simulink model "model_cnn"  (R2020a)
settings: Solver=VariableStepAuto  StartTime=0.0  StopTime=1e6/fs  RelTol=1e-3
PreLoadFcn:
  | setup_imports;
  | %dense2_numerictype = fixdt(1,18,10);
  | %conv1_numerictype = fixdt(1,18,21);
InitFcn:
  | % Intermediate signal dimensions
  | input_dim = [1, 2, 128];
  | layer1_dim = hInterConvLayerDims([1,3,1,64],input_dim,1); % dims : [C,H,W]
  | layer2_dim = hInterConvLayerDims([2,3,64,16],layer1_dim,1);% dims : [C,H,W]
  | layer3_dim = [1,128];
  | 
  | % Conv Layer 1 dimensions
  | conv1_dims = struct(...
  |     'input_dim',    input_dim,...       input_dim = C,H,W
  |     'filter_dim',   [1, 3, 1, 64],...  filter_dim = K,J,C,N
  |     'stride',       1,...
  |     'row_output',   3,...
  |     'output_dim',   layer1_dim);
  | 
  | % Conv Layer 2 dimensions
  | conv2_dims = struct(...
  |     'input_dim',    layer1_dim,...      input = C,H.W
  |     'filter_dim',   [2, 3, 64, 16],...  filter_dim = K,J,C,N
  |     'stride',       1,...
  |     'row_output',   2*3*64,...
  |     'output_dim',   layer2_dim);
  | 
  | % Dense Layer 1 dimensions
  | dense1_dims = struct(...
  |     'input_dim',    layer2_dim,...      input = C,H,W
  |     'weight_dim',   [1984, 128],...     weight_dim = H,W
  |     'output_dim',   layer3_dim);
  | 
  | % Load saved weights and input
  | setup_imports;
  | 
  | fs = 128e6;
  | fs_axi = 100e6;
  | R = 32;
values from neighbouring files (symbols this model uses):
  datatypeInput = X_test.numerictype    [setup_imports.m]
  gemm_wconv1 = fi(hInterleaveFilters(Wconv1),1,16)    [setup_imports.m]
  gemm_wconv2 = fi(hInterleaveFilters(Wconv2),1,16)    [setup_imports.m]
  wdense1 = fi(Wdense1,1,16)    [setup_imports.m]
  wdense2 = fi(Wdense2,1,16)    [setup_imports.m]
undefined symbols (not defined in the file or in its folder): ltehdlRAMinitPO2
libraries: hdlsllib x1022, dspsigops x3, dspsrcs4 x2
(part 3 of 23)

== system model_cnn/HDL CNN Model/Conv Layer 1/Layer 1 Mat-Vec Multiplier/Weight Storage13 ==
  count_Weights : Inport
  Constant : Constant  Value=0  OutDataTypeStr=gemm_wconv1.numerictype  SampleTime=-1
  Constant1 : Constant  Value=false  SampleTime=-1
  Single Port RAM System : hdlsllib/HDL RAMs/Single Port RAM System  RAMType=Single port  WriteOutputValue=New data  RAMInitialValue=[gemm_wconv1(dim,:),zeros(1,4-3)]  SimulateUsing=Code generation
      settings: SourceProductBaseCode=SL
  Out1 : Outport
  wires:
  Single Port RAM System/1 -> Out1/1
  Constant/1 -> Single Port RAM System/1
  Constant1/1 -> Single Port RAM System/3
  count_Weights/1 -> Single Port RAM System/2

== system model_cnn/HDL CNN Model/Conv Layer 1/Layer 1 Mat-Vec Multiplier/Weight Storage14 ==
  count_Weights : Inport
  Constant : Constant  Value=0  OutDataTypeStr=gemm_wconv1.numerictype  SampleTime=-1
  Constant1 : Constant  Value=false  SampleTime=-1
  Single Port RAM System : hdlsllib/HDL RAMs/Single Port RAM System  RAMType=Single port  WriteOutputValue=New data  RAMInitialValue=[gemm_wconv1(dim,:),zeros(1,4-3)]  SimulateUsing=Code generation
      settings: SourceProductBaseCode=SL
  Out1 : Outport
  wires:
  Single Port RAM System/1 -> Out1/1
  Constant/1 -> Single Port RAM System/1
  Constant1/1 -> Single Port RAM System/3
  count_Weights/1 -> Single Port RAM System/2

== system model_cnn/HDL CNN Model/Conv Layer 1/Layer 1 Mat-Vec Multiplier/Weight Storage15 ==
  count_Weights : Inport
  Constant : Constant  Value=0  OutDataTypeStr=gemm_wconv1.numerictype  SampleTime=-1
  Constant1 : Constant  Value=false  SampleTime=-1
  Single Port RAM System : hdlsllib/HDL RAMs/Single Port RAM System  RAMType=Single port  WriteOutputValue=New data  RAMInitialValue=[gemm_wconv1(dim,:),zeros(1,4-3)]  SimulateUsing=Code generation
      settings: SourceProductBaseCode=SL
  Out1 : Outport
  wires:
  Single Port RAM System/1 -> Out1/1
  Constant/1 -> Single Port RAM System/1
  Constant1/1 -> Single Port RAM System/3
  count_Weights/1 -> Single Port RAM System/2

== system model_cnn/HDL CNN Model/Conv Layer 1/Layer 1 Mat-Vec Multiplier/Weight Storage16 ==
  count_Weights : Inport
  Constant : Constant  Value=0  OutDataTypeStr=gemm_wconv1.numerictype  SampleTime=-1
  Constant1 : Constant  Value=false  SampleTime=-1
  Single Port RAM System : hdlsllib/HDL RAMs/Single Port RAM System  RAMType=Single port  WriteOutputValue=New data  RAMInitialValue=[gemm_wconv1(dim,:),zeros(1,4-3)]  SimulateUsing=Code generation
      settings: SourceProductBaseCode=SL
  Out1 : Outport
  wires:
  Single Port RAM System/1 -> Out1/1
  Constant/1 -> Single Port RAM System/1
  Constant1/1 -> Single Port RAM System/3
  count_Weights/1 -> Single Port RAM System/2

== system model_cnn/HDL CNN Model/Conv Layer 1/Layer 1 Mat-Vec Multiplier/Weight Storage17 ==
  count_Weights : Inport
  Constant : Constant  Value=0  OutDataTypeStr=gemm_wconv1.numerictype  SampleTime=-1
  Constant1 : Constant  Value=false  SampleTime=-1
  Single Port RAM System : hdlsllib/HDL RAMs/Single Port RAM System  RAMType=Single port  WriteOutputValue=New data  RAMInitialValue=[gemm_wconv1(dim,:),zeros(1,4-3)]  SimulateUsing=Code generation
      settings: SourceProductBaseCode=SL
  Out1 : Outport
  wires:
  Single Port RAM System/1 -> Out1/1
  Constant/1 -> Single Port RAM System/1
  Constant1/1 -> Single Port RAM System/3
  count_Weights/1 -> Single Port RAM System/2

== system model_cnn/HDL CNN Model/Conv Layer 1/Layer 1 Mat-Vec Multiplier/Weight Storage18 ==
  count_Weights : Inport
  Constant : Constant  Value=0  OutDataTypeStr=gemm_wconv1.numerictype  SampleTime=-1
  Constant1 : Constant  Value=false  SampleTime=-1
  Single Port RAM System : hdlsllib/HDL RAMs/Single Port RAM System  RAMType=Single port  WriteOutputValue=New data  RAMInitialValue=[gemm_wconv1(dim,:),zeros(1,4-3)]  SimulateUsing=Code generation
      settings: SourceProductBaseCode=SL
  Out1 : Outport
  wires:
  Single Port RAM System/1 -> Out1/1
  Constant/1 -> Single Port RAM System/1
  Constant1/1 -> Single Port RAM System/3
  count_Weights/1 -> Single Port RAM System/2

== system model_cnn/HDL CNN Model/Conv Layer 1/Layer 1 Mat-Vec Multiplier/Weight Storage19 ==
  count_Weights : Inport
  Constant : Constant  Value=0  OutDataTypeStr=gemm_wconv1.numerictype  SampleTime=-1
  Constant1 : Constant  Value=false  SampleTime=-1
  Single Port RAM System : hdlsllib/HDL RAMs/Single Port RAM System  RAMType=Single port  WriteOutputValue=New data  RAMInitialValue=[gemm_wconv1(dim,:),zeros(1,4-3)]  SimulateUsing=Code generation
      settings: SourceProductBaseCode=SL
  Out1 : Outport
  wires:
  Single Port RAM System/1 -> Out1/1
  Constant/1 -> Single Port RAM System/1
  Constant1/1 -> Single Port RAM System/3
  count_Weights/1 -> Single Port RAM System/2

== system model_cnn/HDL CNN Model/Conv Layer 1/Layer 1 Mat-Vec Multiplier/Weight Storage2 ==
  count_Weights : Inport
  Constant : Constant  Value=0  OutDataTypeStr=gemm_wconv1.numerictype  SampleTime=-1
  Constant1 : Constant  Value=false  SampleTime=-1
  Single Port RAM System : hdlsllib/HDL RAMs/Single Port RAM System  RAMType=Single port  WriteOutputValue=New data  RAMInitialValue=[gemm_wconv1(dim,:),zeros(1,4-3)]  SimulateUsing=Code generation
      settings: SourceProductBaseCode=SL
  Out1 : Outport
  wires:
  Single Port RAM System/1 -> Out1/1
  Constant/1 -> Single Port RAM System/1
  Constant1/1 -> Single Port RAM System/3
  count_Weights/1 -> Single Port RAM System/2

== system model_cnn/HDL CNN Model/Conv Layer 1/Layer 1 Mat-Vec Multiplier/Weight Storage20 ==
  count_Weights : Inport
  Constant : Constant  Value=0  OutDataTypeStr=gemm_wconv1.numerictype  SampleTime=-1
  Constant1 : Constant  Value=false  SampleTime=-1
  Single Port RAM System : hdlsllib/HDL RAMs/Single Port RAM System  RAMType=Single port  WriteOutputValue=New data  RAMInitialValue=[gemm_wconv1(dim,:),zeros(1,4-3)]  SimulateUsing=Code generation
      settings: SourceProductBaseCode=SL
  Out1 : Outport
  wires:
  Single Port RAM System/1 -> Out1/1
  Constant/1 -> Single Port RAM System/1
  Constant1/1 -> Single Port RAM System/3
  count_Weights/1 -> Single Port RAM System/2

== system model_cnn/HDL CNN Model/Conv Layer 1/Layer 1 Mat-Vec Multiplier/Weight Storage21 ==
  count_Weights : Inport
  Constant : Constant  Value=0  OutDataTypeStr=gemm_wconv1.numerictype  SampleTime=-1
  Constant1 : Constant  Value=false  SampleTime=-1
  Single Port RAM System : hdlsllib/HDL RAMs/Single Port RAM System  RAMType=Single port  WriteOutputValue=New data  RAMInitialValue=[gemm_wconv1(dim,:),zeros(1,4-3)]  SimulateUsing=Code generation
      settings: SourceProductBaseCode=SL
  Out1 : Outport
  wires:
  Single Port RAM System/1 -> Out1/1
  Constant/1 -> Single Port RAM System/1
  Constant1/1 -> Single Port RAM System/3
  count_Weights/1 -> Single Port RAM System/2

== system model_cnn/HDL CNN Model/Conv Layer 1/Layer 1 Mat-Vec Multiplier/Weight Storage22 ==
  count_Weights : Inport
  Constant : Constant  Value=0  OutDataTypeStr=gemm_wconv1.numerictype  SampleTime=-1
  Constant1 : Constant  Value=false  SampleTime=-1
  Single Port RAM System : hdlsllib/HDL RAMs/Single Port RAM System  RAMType=Single port  WriteOutputValue=New data  RAMInitialValue=[gemm_wconv1(dim,:),zeros(1,4-3)]  SimulateUsing=Code generation
      settings: SourceProductBaseCode=SL
  Out1 : Outport
  wires:
  Single Port RAM System/1 -> Out1/1
  Constant/1 -> Single Port RAM System/1
  Constant1/1 -> Single Port RAM System/3
  count_Weights/1 -> Single Port RAM System/2

== system model_cnn/HDL CNN Model/Conv Layer 1/Layer 1 Mat-Vec Multiplier/Weight Storage23 ==
  count_Weights : Inport
  Constant : Constant  Value=0  OutDataTypeStr=gemm_wconv1.numerictype  SampleTime=-1
  Constant1 : Constant  Value=false  SampleTime=-1
  Single Port RAM System : hdlsllib/HDL RAMs/Single Port RAM System  RAMType=Single port  WriteOutputValue=New data  RAMInitialValue=[gemm_wconv1(dim,:),zeros(1,4-3)]  SimulateUsing=Code generation
      settings: SourceProductBaseCode=SL
  Out1 : Outport
  wires:
  Single Port RAM System/1 -> Out1/1
  Constant/1 -> Single Port RAM System/1
  Constant1/1 -> Single Port RAM System/3
  count_Weights/1 -> Single Port RAM System/2

== system model_cnn/HDL CNN Model/Conv Layer 1/Layer 1 Mat-Vec Multiplier/Weight Storage24 ==
  count_Weights : Inport
  Constant : Constant  Value=0  OutDataTypeStr=gemm_wconv1.numerictype  SampleTime=-1
  Constant1 : Constant  Value=false  SampleTime=-1
  Single Port RAM System : hdlsllib/HDL RAMs/Single Port RAM System  RAMType=Single port  WriteOutputValue=New data  RAMInitialValue=[gemm_wconv1(dim,:),zeros(1,4-3)]  SimulateUsing=Code generation
      settings: SourceProductBaseCode=SL
  Out1 : Outport
  wires:
  Single Port RAM System/1 -> Out1/1
  Constant/1 -> Single Port RAM System/1
  Constant1/1 -> Single Port RAM System/3
  count_Weights/1 -> Single Port RAM System/2

== system model_cnn/HDL CNN Model/Conv Layer 1/Layer 1 Mat-Vec Multiplier/Weight Storage25 ==
  count_Weights : Inport
  Constant : Constant  Value=0  OutDataTypeStr=gemm_wconv1.numerictype  SampleTime=-1
  Constant1 : Constant  Value=false  SampleTime=-1
  Single Port RAM System : hdlsllib/HDL RAMs/Single Port RAM System  RAMType=Single port  WriteOutputValue=New data  RAMInitialValue=[gemm_wconv1(dim,:),zeros(1,4-3)]  SimulateUsing=Code generation
      settings: SourceProductBaseCode=SL
  Out1 : Outport
  wires:
  Single Port RAM System/1 -> Out1/1
  Constant/1 -> Single Port RAM System/1
  Constant1/1 -> Single Port RAM System/3
  count_Weights/1 -> Single Port RAM System/2

== system model_cnn/HDL CNN Model/Conv Layer 1/Layer 1 Mat-Vec Multiplier/Weight Storage26 ==
  count_Weights : Inport
  Constant : Constant  Value=0  OutDataTypeStr=gemm_wconv1.numerictype  SampleTime=-1
  Constant1 : Constant  Value=false  SampleTime=-1
  Single Port RAM System : hdlsllib/HDL RAMs/Single Port RAM System  RAMType=Single port  WriteOutputValue=New data  RAMInitialValue=[gemm_wconv1(dim,:),zeros(1,4-3)]  SimulateUsing=Code generation
      settings: SourceProductBaseCode=SL
  Out1 : Outport
  wires:
  Single Port RAM System/1 -> Out1/1
  Constant/1 -> Single Port RAM System/1
  Constant1/1 -> Single Port RAM System/3
  count_Weights/1 -> Single Port RAM System/2

== system model_cnn/HDL CNN Model/Conv Layer 1/Layer 1 Mat-Vec Multiplier/Weight Storage27 ==
  count_Weights : Inport
  Constant : Constant  Value=0  OutDataTypeStr=gemm_wconv1.numerictype  SampleTime=-1
  Constant1 : Constant  Value=false  SampleTime=-1
  Single Port RAM System : hdlsllib/HDL RAMs/Single Port RAM System  RAMType=Single port  WriteOutputValue=New data  RAMInitialValue=[gemm_wconv1(dim,:),zeros(1,4-3)]  SimulateUsing=Code generation
      settings: SourceProductBaseCode=SL
  Out1 : Outport
  wires:
  Single Port RAM System/1 -> Out1/1
  Constant/1 -> Single Port RAM System/1
  Constant1/1 -> Single Port RAM System/3
  count_Weights/1 -> Single Port RAM System/2

== system model_cnn/HDL CNN Model/Conv Layer 1/Layer 1 Mat-Vec Multiplier/Weight Storage28 ==
  count_Weights : Inport
  Constant : Constant  Value=0  OutDataTypeStr=gemm_wconv1.numerictype  SampleTime=-1
  Constant1 : Constant  Value=false  SampleTime=-1
  Single Port RAM System : hdlsllib/HDL RAMs/Single Port RAM System  RAMType=Single port  WriteOutputValue=New data  RAMInitialValue=[gemm_wconv1(dim,:),zeros(1,4-3)]  SimulateUsing=Code generation
      settings: SourceProductBaseCode=SL
  Out1 : Outport
  wires:
  Single Port RAM System/1 -> Out1/1
  Constant/1 -> Single Port RAM System/1
  Constant1/1 -> Single Port RAM System/3
  count_Weights/1 -> Single Port RAM System/2

== system model_cnn/HDL CNN Model/Conv Layer 1/Layer 1 Mat-Vec Multiplier/Weight Storage29 ==
  count_Weights : Inport
  Constant : Constant  Value=0  OutDataTypeStr=gemm_wconv1.numerictype  SampleTime=-1
  Constant1 : Constant  Value=false  SampleTime=-1
  Single Port RAM System : hdlsllib/HDL RAMs/Single Port RAM System  RAMType=Single port  WriteOutputValue=New data  RAMInitialValue=[gemm_wconv1(dim,:),zeros(1,4-3)]  SimulateUsing=Code generation
      settings: SourceProductBaseCode=SL
  Out1 : Outport
  wires:
  Single Port RAM System/1 -> Out1/1
  Constant/1 -> Single Port RAM System/1
  Constant1/1 -> Single Port RAM System/3
  count_Weights/1 -> Single Port RAM System/2

== system model_cnn/HDL CNN Model/Conv Layer 1/Layer 1 Mat-Vec Multiplier/Weight Storage3 ==
  count_Weights : Inport
  Constant : Constant  Value=0  OutDataTypeStr=gemm_wconv1.numerictype  SampleTime=-1
  Constant1 : Constant  Value=false  SampleTime=-1
  Single Port RAM System : hdlsllib/HDL RAMs/Single Port RAM System  RAMType=Single port  WriteOutputValue=New data  RAMInitialValue=[gemm_wconv1(dim,:),zeros(1,4-3)]  SimulateUsing=Code generation
      settings: SourceProductBaseCode=SL
  Out1 : Outport
  wires:
  Single Port RAM System/1 -> Out1/1
  Constant/1 -> Single Port RAM System/1
  Constant1/1 -> Single Port RAM System/3
  count_Weights/1 -> Single Port RAM System/2

== system model_cnn/HDL CNN Model/Conv Layer 1/Layer 1 Mat-Vec Multiplier/Weight Storage30 ==
  count_Weights : Inport
  Constant : Constant  Value=0  OutDataTypeStr=gemm_wconv1.numerictype  SampleTime=-1
  Constant1 : Constant  Value=false  SampleTime=-1
  Single Port RAM System : hdlsllib/HDL RAMs/Single Port RAM System  RAMType=Single port  WriteOutputValue=New data  RAMInitialValue=[gemm_wconv1(dim,:),zeros(1,4-3)]  SimulateUsing=Code generation
      settings: SourceProductBaseCode=SL
  Out1 : Outport
  wires:
  Single Port RAM System/1 -> Out1/1
  Constant/1 -> Single Port RAM System/1
  Constant1/1 -> Single Port RAM System/3
  count_Weights/1 -> Single Port RAM System/2

== system model_cnn/HDL CNN Model/Conv Layer 1/Layer 1 Mat-Vec Multiplier/Weight Storage31 ==
  count_Weights : Inport
  Constant : Constant  Value=0  OutDataTypeStr=gemm_wconv1.numerictype  SampleTime=-1
  Constant1 : Constant  Value=false  SampleTime=-1
  Single Port RAM System : hdlsllib/HDL RAMs/Single Port RAM System  RAMType=Single port  WriteOutputValue=New data  RAMInitialValue=[gemm_wconv1(dim,:),zeros(1,4-3)]  SimulateUsing=Code generation
      settings: SourceProductBaseCode=SL
  Out1 : Outport
  wires:
  Single Port RAM System/1 -> Out1/1
  Constant/1 -> Single Port RAM System/1
  Constant1/1 -> Single Port RAM System/3
  count_Weights/1 -> Single Port RAM System/2

== system model_cnn/HDL CNN Model/Conv Layer 1/Layer 1 Mat-Vec Multiplier/Weight Storage32 ==
  count_Weights : Inport
  Constant : Constant  Value=0  OutDataTypeStr=gemm_wconv1.numerictype  SampleTime=-1
  Constant1 : Constant  Value=false  SampleTime=-1
  Single Port RAM System : hdlsllib/HDL RAMs/Single Port RAM System  RAMType=Single port  WriteOutputValue=New data  RAMInitialValue=[gemm_wconv1(dim,:),zeros(1,4-3)]  SimulateUsing=Code generation
      settings: SourceProductBaseCode=SL
  Out1 : Outport
  wires:
  Single Port RAM System/1 -> Out1/1
  Constant/1 -> Single Port RAM System/1
  Constant1/1 -> Single Port RAM System/3
  count_Weights/1 -> Single Port RAM System/2

== system model_cnn/HDL CNN Model/Conv Layer 1/Layer 1 Mat-Vec Multiplier/Weight Storage33 ==
  count_Weights : Inport
  Constant : Constant  Value=0  OutDataTypeStr=gemm_wconv1.numerictype  SampleTime=-1
  Constant1 : Constant  Value=false  SampleTime=-1
  Single Port RAM System : hdlsllib/HDL RAMs/Single Port RAM System  RAMType=Single port  WriteOutputValue=New data  RAMInitialValue=[gemm_wconv1(dim,:),zeros(1,4-3)]  SimulateUsing=Code generation
      settings: SourceProductBaseCode=SL
  Out1 : Outport
  wires:
  Single Port RAM System/1 -> Out1/1
  Constant/1 -> Single Port RAM System/1
  Constant1/1 -> Single Port RAM System/3
  count_Weights/1 -> Single Port RAM System/2

== system model_cnn/HDL CNN Model/Conv Layer 1/Layer 1 Mat-Vec Multiplier/Weight Storage34 ==
  count_Weights : Inport
  Constant : Constant  Value=0  OutDataTypeStr=gemm_wconv1.numerictype  SampleTime=-1
  Constant1 : Constant  Value=false  SampleTime=-1
  Single Port RAM System : hdlsllib/HDL RAMs/Single Port RAM System  RAMType=Single port  WriteOutputValue=New data  RAMInitialValue=[gemm_wconv1(dim,:),zeros(1,4-3)]  SimulateUsing=Code generation
      settings: SourceProductBaseCode=SL
  Out1 : Outport
  wires:
  Single Port RAM System/1 -> Out1/1
  Constant/1 -> Single Port RAM System/1
  Constant1/1 -> Single Port RAM System/3
  count_Weights/1 -> Single Port RAM System/2

== system model_cnn/HDL CNN Model/Conv Layer 1/Layer 1 Mat-Vec Multiplier/Weight Storage35 ==
  count_Weights : Inport
  Constant : Constant  Value=0  OutDataTypeStr=gemm_wconv1.numerictype  SampleTime=-1
  Constant1 : Constant  Value=false  SampleTime=-1
  Single Port RAM System : hdlsllib/HDL RAMs/Single Port RAM System  RAMType=Single port  WriteOutputValue=New data  RAMInitialValue=[gemm_wconv1(dim,:),zeros(1,4-3)]  SimulateUsing=Code generation
      settings: SourceProductBaseCode=SL
  Out1 : Outport
  wires:
  Single Port RAM System/1 -> Out1/1
  Constant/1 -> Single Port RAM System/1
  Constant1/1 -> Single Port RAM System/3
  count_Weights/1 -> Single Port RAM System/2

== system model_cnn/HDL CNN Model/Conv Layer 1/Layer 1 Mat-Vec Multiplier/Weight Storage36 ==
  count_Weights : Inport
  Constant : Constant  Value=0  OutDataTypeStr=gemm_wconv1.numerictype  SampleTime=-1
  Constant1 : Constant  Value=false  SampleTime=-1
  Single Port RAM System : hdlsllib/HDL RAMs/Single Port RAM System  RAMType=Single port  WriteOutputValue=New data  RAMInitialValue=[gemm_wconv1(dim,:),zeros(1,4-3)]  SimulateUsing=Code generation
      settings: SourceProductBaseCode=SL
  Out1 : Outport
  wires:
  Single Port RAM System/1 -> Out1/1
  Constant/1 -> Single Port RAM System/1
  Constant1/1 -> Single Port RAM System/3
  count_Weights/1 -> Single Port RAM System/2

== system model_cnn/HDL CNN Model/Conv Layer 1/Layer 1 Mat-Vec Multiplier/Weight Storage37 ==
  count_Weights : Inport
  Constant : Constant  Value=0  OutDataTypeStr=gemm_wconv1.numerictype  SampleTime=-1
  Constant1 : Constant  Value=false  SampleTime=-1
  Single Port RAM System : hdlsllib/HDL RAMs/Single Port RAM System  RAMType=Single port  WriteOutputValue=New data  RAMInitialValue=[gemm_wconv1(dim,:),zeros(1,4-3)]  SimulateUsing=Code generation
      settings: SourceProductBaseCode=SL
  Out1 : Outport
  wires:
  Single Port RAM System/1 -> Out1/1
  Constant/1 -> Single Port RAM System/1
  Constant1/1 -> Single Port RAM System/3
  count_Weights/1 -> Single Port RAM System/2

== system model_cnn/HDL CNN Model/Conv Layer 1/Layer 1 Mat-Vec Multiplier/Weight Storage38 ==
  count_Weights : Inport
  Constant : Constant  Value=0  OutDataTypeStr=gemm_wconv1.numerictype  SampleTime=-1
  Constant1 : Constant  Value=false  SampleTime=-1
  Single Port RAM System : hdlsllib/HDL RAMs/Single Port RAM System  RAMType=Single port  WriteOutputValue=New data  RAMInitialValue=[gemm_wconv1(dim,:),zeros(1,4-3)]  SimulateUsing=Code generation
      settings: SourceProductBaseCode=SL
  Out1 : Outport
  wires:
  Single Port RAM System/1 -> Out1/1
  Constant/1 -> Single Port RAM System/1
  Constant1/1 -> Single Port RAM System/3
  count_Weights/1 -> Single Port RAM System/2

== system model_cnn/HDL CNN Model/Conv Layer 1/Layer 1 Mat-Vec Multiplier/Weight Storage39 ==
  count_Weights : Inport
  Constant : Constant  Value=0  OutDataTypeStr=gemm_wconv1.numerictype  SampleTime=-1
  Constant1 : Constant  Value=false  SampleTime=-1
  Single Port RAM System : hdlsllib/HDL RAMs/Single Port RAM System  RAMType=Single port  WriteOutputValue=New data  RAMInitialValue=[gemm_wconv1(dim,:),zeros(1,4-3)]  SimulateUsing=Code generation
      settings: SourceProductBaseCode=SL
  Out1 : Outport
  wires:
  Single Port RAM System/1 -> Out1/1
  Constant/1 -> Single Port RAM System/1
  Constant1/1 -> Single Port RAM System/3
  count_Weights/1 -> Single Port RAM System/2

== system model_cnn/HDL CNN Model/Conv Layer 1/Layer 1 Mat-Vec Multiplier/Weight Storage4 ==
  count_Weights : Inport
  Constant : Constant  Value=0  OutDataTypeStr=gemm_wconv1.numerictype  SampleTime=-1
  Constant1 : Constant  Value=false  SampleTime=-1
  Single Port RAM System : hdlsllib/HDL RAMs/Single Port RAM System  RAMType=Single port  WriteOutputValue=New data  RAMInitialValue=[gemm_wconv1(dim,:),zeros(1,4-3)]  SimulateUsing=Code generation
      settings: SourceProductBaseCode=SL
  Out1 : Outport
  wires:
  Single Port RAM System/1 -> Out1/1
  Constant/1 -> Single Port RAM System/1
  Constant1/1 -> Single Port RAM System/3
  count_Weights/1 -> Single Port RAM System/2

== system model_cnn/HDL CNN Model/Conv Layer 1/Layer 1 Mat-Vec Multiplier/Weight Storage40 ==
  count_Weights : Inport
  Constant : Constant  Value=0  OutDataTypeStr=gemm_wconv1.numerictype  SampleTime=-1
  Constant1 : Constant  Value=false  SampleTime=-1
  Single Port RAM System : hdlsllib/HDL RAMs/Single Port RAM System  RAMType=Single port  WriteOutputValue=New data  RAMInitialValue=[gemm_wconv1(dim,:),zeros(1,4-3)]  SimulateUsing=Code generation
      settings: SourceProductBaseCode=SL
  Out1 : Outport
  wires:
  Single Port RAM System/1 -> Out1/1
  Constant/1 -> Single Port RAM System/1
  Constant1/1 -> Single Port RAM System/3
  count_Weights/1 -> Single Port RAM System/2

== system model_cnn/HDL CNN Model/Conv Layer 1/Layer 1 Mat-Vec Multiplier/Weight Storage41 ==
  count_Weights : Inport
  Constant : Constant  Value=0  OutDataTypeStr=gemm_wconv1.numerictype  SampleTime=-1
  Constant1 : Constant  Value=false  SampleTime=-1
  Single Port RAM System : hdlsllib/HDL RAMs/Single Port RAM System  RAMType=Single port  WriteOutputValue=New data  RAMInitialValue=[gemm_wconv1(dim,:),zeros(1,4-3)]  SimulateUsing=Code generation
      settings: SourceProductBaseCode=SL
  Out1 : Outport
  wires:
  Single Port RAM System/1 -> Out1/1
  Constant/1 -> Single Port RAM System/1
  Constant1/1 -> Single Port RAM System/3
  count_Weights/1 -> Single Port RAM System/2

== system model_cnn/HDL CNN Model/Conv Layer 1/Layer 1 Mat-Vec Multiplier/Weight Storage42 ==
  count_Weights : Inport
  Constant : Constant  Value=0  OutDataTypeStr=gemm_wconv1.numerictype  SampleTime=-1
  Constant1 : Constant  Value=false  SampleTime=-1
  Single Port RAM System : hdlsllib/HDL RAMs/Single Port RAM System  RAMType=Single port  WriteOutputValue=New data  RAMInitialValue=[gemm_wconv1(dim,:),zeros(1,4-3)]  SimulateUsing=Code generation
      settings: SourceProductBaseCode=SL
  Out1 : Outport
  wires:
  Single Port RAM System/1 -> Out1/1
  Constant/1 -> Single Port RAM System/1
  Constant1/1 -> Single Port RAM System/3
  count_Weights/1 -> Single Port RAM System/2

== system model_cnn/HDL CNN Model/Conv Layer 1/Layer 1 Mat-Vec Multiplier/Weight Storage43 ==
  count_Weights : Inport
  Constant : Constant  Value=0  OutDataTypeStr=gemm_wconv1.numerictype  SampleTime=-1
  Constant1 : Constant  Value=false  SampleTime=-1
  Single Port RAM System : hdlsllib/HDL RAMs/Single Port RAM System  RAMType=Single port  WriteOutputValue=New data  RAMInitialValue=[gemm_wconv1(dim,:),zeros(1,4-3)]  SimulateUsing=Code generation
      settings: SourceProductBaseCode=SL
  Out1 : Outport
  wires:
  Single Port RAM System/1 -> Out1/1
  Constant/1 -> Single Port RAM System/1
  Constant1/1 -> Single Port RAM System/3
  count_Weights/1 -> Single Port RAM System/2

== system model_cnn/HDL CNN Model/Conv Layer 1/Layer 1 Mat-Vec Multiplier/Weight Storage44 ==
  count_Weights : Inport
  Constant : Constant  Value=0  OutDataTypeStr=gemm_wconv1.numerictype  SampleTime=-1
  Constant1 : Constant  Value=false  SampleTime=-1
  Single Port RAM System : hdlsllib/HDL RAMs/Single Port RAM System  RAMType=Single port  WriteOutputValue=New data  RAMInitialValue=[gemm_wconv1(dim,:),zeros(1,4-3)]  SimulateUsing=Code generation
      settings: SourceProductBaseCode=SL
  Out1 : Outport
  wires:
  Single Port RAM System/1 -> Out1/1
  Constant/1 -> Single Port RAM System/1
  Constant1/1 -> Single Port RAM System/3
  count_Weights/1 -> Single Port RAM System/2

== system model_cnn/HDL CNN Model/Conv Layer 1/Layer 1 Mat-Vec Multiplier/Weight Storage45 ==
  count_Weights : Inport
  Constant : Constant  Value=0  OutDataTypeStr=gemm_wconv1.numerictype  SampleTime=-1
  Constant1 : Constant  Value=false  SampleTime=-1
  Single Port RAM System : hdlsllib/HDL RAMs/Single Port RAM System  RAMType=Single port  WriteOutputValue=New data  RAMInitialValue=[gemm_wconv1(dim,:),zeros(1,4-3)]  SimulateUsing=Code generation
      settings: SourceProductBaseCode=SL
  Out1 : Outport
  wires:
  Single Port RAM System/1 -> Out1/1
  Constant/1 -> Single Port RAM System/1
  Constant1/1 -> Single Port RAM System/3
  count_Weights/1 -> Single Port RAM System/2

== system model_cnn/HDL CNN Model/Conv Layer 1/Layer 1 Mat-Vec Multiplier/Weight Storage46 ==
  count_Weights : Inport
  Constant : Constant  Value=0  OutDataTypeStr=gemm_wconv1.numerictype  SampleTime=-1
  Constant1 : Constant  Value=false  SampleTime=-1
  Single Port RAM System : hdlsllib/HDL RAMs/Single Port RAM System  RAMType=Single port  WriteOutputValue=New data  RAMInitialValue=[gemm_wconv1(dim,:),zeros(1,4-3)]  SimulateUsing=Code generation
      settings: SourceProductBaseCode=SL
  Out1 : Outport
  wires:
  Single Port RAM System/1 -> Out1/1
  Constant/1 -> Single Port RAM System/1
  Constant1/1 -> Single Port RAM System/3
  count_Weights/1 -> Single Port RAM System/2

== system model_cnn/HDL CNN Model/Conv Layer 1/Layer 1 Mat-Vec Multiplier/Weight Storage47 ==
  count_Weights : Inport
  Constant : Constant  Value=0  OutDataTypeStr=gemm_wconv1.numerictype  SampleTime=-1
  Constant1 : Constant  Value=false  SampleTime=-1
  Single Port RAM System : hdlsllib/HDL RAMs/Single Port RAM System  RAMType=Single port  WriteOutputValue=New data  RAMInitialValue=[gemm_wconv1(dim,:),zeros(1,4-3)]  SimulateUsing=Code generation
      settings: SourceProductBaseCode=SL
  Out1 : Outport
  wires:
  Single Port RAM System/1 -> Out1/1
  Constant/1 -> Single Port RAM System/1
  Constant1/1 -> Single Port RAM System/3
  count_Weights/1 -> Single Port RAM System/2

== system model_cnn/HDL CNN Model/Conv Layer 1/Layer 1 Mat-Vec Multiplier/Weight Storage48 ==
  count_Weights : Inport
  Constant : Constant  Value=0  OutDataTypeStr=gemm_wconv1.numerictype  SampleTime=-1
  Constant1 : Constant  Value=false  SampleTime=-1
  Single Port RAM System : hdlsllib/HDL RAMs/Single Port RAM System  RAMType=Single port  WriteOutputValue=New data  RAMInitialValue=[gemm_wconv1(dim,:),zeros(1,4-3)]  SimulateUsing=Code generation
      settings: SourceProductBaseCode=SL
  Out1 : Outport
  wires:
  Single Port RAM System/1 -> Out1/1
  Constant/1 -> Single Port RAM System/1
  Constant1/1 -> Single Port RAM System/3
  count_Weights/1 -> Single Port RAM System/2

== system model_cnn/HDL CNN Model/Conv Layer 1/Layer 1 Mat-Vec Multiplier/Weight Storage49 ==
  count_Weights : Inport
  Constant : Constant  Value=0  OutDataTypeStr=gemm_wconv1.numerictype  SampleTime=-1
  Constant1 : Constant  Value=false  SampleTime=-1
  Single Port RAM System : hdlsllib/HDL RAMs/Single Port RAM System  RAMType=Single port  WriteOutputValue=New data  RAMInitialValue=[gemm_wconv1(dim,:),zeros(1,4-3)]  SimulateUsing=Code generation
      settings: SourceProductBaseCode=SL
  Out1 : Outport
  wires:
  Single Port RAM System/1 -> Out1/1
  Constant/1 -> Single Port RAM System/1
  Constant1/1 -> Single Port RAM System/3
  count_Weights/1 -> Single Port RAM System/2

== system model_cnn/HDL CNN Model/Conv Layer 1/Layer 1 Mat-Vec Multiplier/Weight Storage5 ==
  count_Weights : Inport
  Constant : Constant  Value=0  OutDataTypeStr=gemm_wconv1.numerictype  SampleTime=-1
  Constant1 : Constant  Value=false  SampleTime=-1
  Single Port RAM System : hdlsllib/HDL RAMs/Single Port RAM System  RAMType=Single port  WriteOutputValue=New data  RAMInitialValue=[gemm_wconv1(dim,:),zeros(1,4-3)]  SimulateUsing=Code generation
      settings: SourceProductBaseCode=SL
  Out1 : Outport
  wires:
  Single Port RAM System/1 -> Out1/1
  Constant/1 -> Single Port RAM System/1
  Constant1/1 -> Single Port RAM System/3
  count_Weights/1 -> Single Port RAM System/2

== system model_cnn/HDL CNN Model/Conv Layer 1/Layer 1 Mat-Vec Multiplier/Weight Storage50 ==
  count_Weights : Inport
  Constant : Constant  Value=0  OutDataTypeStr=gemm_wconv1.numerictype  SampleTime=-1
  Constant1 : Constant  Value=false  SampleTime=-1
  Single Port RAM System : hdlsllib/HDL RAMs/Single Port RAM System  RAMType=Single port  WriteOutputValue=New data  RAMInitialValue=[gemm_wconv1(dim,:),zeros(1,4-3)]  SimulateUsing=Code generation
      settings: SourceProductBaseCode=SL
  Out1 : Outport
  wires:
  Single Port RAM System/1 -> Out1/1
  Constant/1 -> Single Port RAM System/1
  Constant1/1 -> Single Port RAM System/3
  count_Weights/1 -> Single Port RAM System/2

== system model_cnn/HDL CNN Model/Conv Layer 1/Layer 1 Mat-Vec Multiplier/Weight Storage51 ==
  count_Weights : Inport
  Constant : Constant  Value=0  OutDataTypeStr=gemm_wconv1.numerictype  SampleTime=-1
  Constant1 : Constant  Value=false  SampleTime=-1
  Single Port RAM System : hdlsllib/HDL RAMs/Single Port RAM System  RAMType=Single port  WriteOutputValue=New data  RAMInitialValue=[gemm_wconv1(dim,:),zeros(1,4-3)]  SimulateUsing=Code generation
      settings: SourceProductBaseCode=SL
  Out1 : Outport
  wires:
  Single Port RAM System/1 -> Out1/1
  Constant/1 -> Single Port RAM System/1
  Constant1/1 -> Single Port RAM System/3
  count_Weights/1 -> Single Port RAM System/2

== system model_cnn/HDL CNN Model/Conv Layer 1/Layer 1 Mat-Vec Multiplier/Weight Storage52 ==
  count_Weights : Inport
  Constant : Constant  Value=0  OutDataTypeStr=gemm_wconv1.numerictype  SampleTime=-1
  Constant1 : Constant  Value=false  SampleTime=-1
  Single Port RAM System : hdlsllib/HDL RAMs/Single Port RAM System  RAMType=Single port  WriteOutputValue=New data  RAMInitialValue=[gemm_wconv1(dim,:),zeros(1,4-3)]  SimulateUsing=Code generation
      settings: SourceProductBaseCode=SL
  Out1 : Outport
  wires:
  Single Port RAM System/1 -> Out1/1
  Constant/1 -> Single Port RAM System/1
  Constant1/1 -> Single Port RAM System/3
  count_Weights/1 -> Single Port RAM System/2

== system model_cnn/HDL CNN Model/Conv Layer 1/Layer 1 Mat-Vec Multiplier/Weight Storage53 ==
  count_Weights : Inport
  Constant : Constant  Value=0  OutDataTypeStr=gemm_wconv1.numerictype  SampleTime=-1
  Constant1 : Constant  Value=false  SampleTime=-1
  Single Port RAM System : hdlsllib/HDL RAMs/Single Port RAM System  RAMType=Single port  WriteOutputValue=New data  RAMInitialValue=[gemm_wconv1(dim,:),zeros(1,4-3)]  SimulateUsing=Code generation
      settings: SourceProductBaseCode=SL
  Out1 : Outport
  wires:
  Single Port RAM System/1 -> Out1/1
  Constant/1 -> Single Port RAM System/1
  Constant1/1 -> Single Port RAM System/3
  count_Weights/1 -> Single Port RAM System/2

== system model_cnn/HDL CNN Model/Conv Layer 1/Layer 1 Mat-Vec Multiplier/Weight Storage54 ==
  count_Weights : Inport
  Constant : Constant  Value=0  OutDataTypeStr=gemm_wconv1.numerictype  SampleTime=-1
  Constant1 : Constant  Value=false  SampleTime=-1
  Single Port RAM System : hdlsllib/HDL RAMs/Single Port RAM System  RAMType=Single port  WriteOutputValue=New data  RAMInitialValue=[gemm_wconv1(dim,:),zeros(1,4-3)]  SimulateUsing=Code generation
      settings: SourceProductBaseCode=SL
  Out1 : Outport
  wires:
  Single Port RAM System/1 -> Out1/1
  Constant/1 -> Single Port RAM System/1
  Constant1/1 -> Single Port RAM System/3
  count_Weights/1 -> Single Port RAM System/2

== system model_cnn/HDL CNN Model/Conv Layer 1/Layer 1 Mat-Vec Multiplier/Weight Storage55 ==
  count_Weights : Inport
  Constant : Constant  Value=0  OutDataTypeStr=gemm_wconv1.numerictype  SampleTime=-1
  Constant1 : Constant  Value=false  SampleTime=-1
  Single Port RAM System : hdlsllib/HDL RAMs/Single Port RAM System  RAMType=Single port  WriteOutputValue=New data  RAMInitialValue=[gemm_wconv1(dim,:),zeros(1,4-3)]  SimulateUsing=Code generation
      settings: SourceProductBaseCode=SL
  Out1 : Outport
  wires:
  Single Port RAM System/1 -> Out1/1
  Constant/1 -> Single Port RAM System/1
  Constant1/1 -> Single Port RAM System/3
  count_Weights/1 -> Single Port RAM System/2

== system model_cnn/HDL CNN Model/Conv Layer 1/Layer 1 Mat-Vec Multiplier/Weight Storage56 ==
  count_Weights : Inport
  Constant : Constant  Value=0  OutDataTypeStr=gemm_wconv1.numerictype  SampleTime=-1
  Constant1 : Constant  Value=false  SampleTime=-1
  Single Port RAM System : hdlsllib/HDL RAMs/Single Port RAM System  RAMType=Single port  WriteOutputValue=New data  RAMInitialValue=[gemm_wconv1(dim,:),zeros(1,4-3)]  SimulateUsing=Code generation
      settings: SourceProductBaseCode=SL
  Out1 : Outport
  wires:
  Single Port RAM System/1 -> Out1/1
  Constant/1 -> Single Port RAM System/1
  Constant1/1 -> Single Port RAM System/3
  count_Weights/1 -> Single Port RAM System/2

== system model_cnn/HDL CNN Model/Conv Layer 1/Layer 1 Mat-Vec Multiplier/Weight Storage57 ==
  count_Weights : Inport
  Constant : Constant  Value=0  OutDataTypeStr=gemm_wconv1.numerictype  SampleTime=-1
  Constant1 : Constant  Value=false  SampleTime=-1
  Single Port RAM System : hdlsllib/HDL RAMs/Single Port RAM System  RAMType=Single port  WriteOutputValue=New data  RAMInitialValue=[gemm_wconv1(dim,:),zeros(1,4-3)]  SimulateUsing=Code generation
      settings: SourceProductBaseCode=SL
  Out1 : Outport
  wires:
  Single Port RAM System/1 -> Out1/1
  Constant/1 -> Single Port RAM System/1
  Constant1/1 -> Single Port RAM System/3
  count_Weights/1 -> Single Port RAM System/2

== system model_cnn/HDL CNN Model/Conv Layer 1/Layer 1 Mat-Vec Multiplier/Weight Storage58 ==
  count_Weights : Inport
  Constant : Constant  Value=0  OutDataTypeStr=gemm_wconv1.numerictype  SampleTime=-1
  Constant1 : Constant  Value=false  SampleTime=-1
  Single Port RAM System : hdlsllib/HDL RAMs/Single Port RAM System  RAMType=Single port  WriteOutputValue=New data  RAMInitialValue=[gemm_wconv1(dim,:),zeros(1,4-3)]  SimulateUsing=Code generation
      settings: SourceProductBaseCode=SL
  Out1 : Outport
  wires:
  Single Port RAM System/1 -> Out1/1
  Constant/1 -> Single Port RAM System/1
  Constant1/1 -> Single Port RAM System/3
  count_Weights/1 -> Single Port RAM System/2

== system model_cnn/HDL CNN Model/Conv Layer 1/Layer 1 Mat-Vec Multiplier/Weight Storage59 ==
  count_Weights : Inport
  Constant : Constant  Value=0  OutDataTypeStr=gemm_wconv1.numerictype  SampleTime=-1
  Constant1 : Constant  Value=false  SampleTime=-1
  Single Port RAM System : hdlsllib/HDL RAMs/Single Port RAM System  RAMType=Single port  WriteOutputValue=New data  RAMInitialValue=[gemm_wconv1(dim,:),zeros(1,4-3)]  SimulateUsing=Code generation
      settings: SourceProductBaseCode=SL
  Out1 : Outport
  wires:
  Single Port RAM System/1 -> Out1/1
  Constant/1 -> Single Port RAM System/1
  Constant1/1 -> Single Port RAM System/3
  count_Weights/1 -> Single Port RAM System/2

== system model_cnn/HDL CNN Model/Conv Layer 1/Layer 1 Mat-Vec Multiplier/Weight Storage6 ==
  count_Weights : Inport
  Constant : Constant  Value=0  OutDataTypeStr=gemm_wconv1.numerictype  SampleTime=-1
  Constant1 : Constant  Value=false  SampleTime=-1
  Single Port RAM System : hdlsllib/HDL RAMs/Single Port RAM System  RAMType=Single port  WriteOutputValue=New data  RAMInitialValue=[gemm_wconv1(dim,:),zeros(1,4-3)]  SimulateUsing=Code generation
      settings: SourceProductBaseCode=SL
  Out1 : Outport
  wires:
  Single Port RAM System/1 -> Out1/1
  Constant/1 -> Single Port RAM System/1
  Constant1/1 -> Single Port RAM System/3
  count_Weights/1 -> Single Port RAM System/2

== system model_cnn/HDL CNN Model/Conv Layer 1/Layer 1 Mat-Vec Multiplier/Weight Storage60 ==
  count_Weights : Inport
  Constant : Constant  Value=0  OutDataTypeStr=gemm_wconv1.numerictype  SampleTime=-1
  Constant1 : Constant  Value=false  SampleTime=-1
  Single Port RAM System : hdlsllib/HDL RAMs/Single Port RAM System  RAMType=Single port  WriteOutputValue=New data  RAMInitialValue=[gemm_wconv1(dim,:),zeros(1,4-3)]  SimulateUsing=Code generation
      settings: SourceProductBaseCode=SL
  Out1 : Outport
  wires:
  Single Port RAM System/1 -> Out1/1
  Constant/1 -> Single Port RAM System/1
  Constant1/1 -> Single Port RAM System/3
  count_Weights/1 -> Single Port RAM System/2

== system model_cnn/HDL CNN Model/Conv Layer 1/Layer 1 Mat-Vec Multiplier/Weight Storage61 ==
  count_Weights : Inport
  Constant : Constant  Value=0  OutDataTypeStr=gemm_wconv1.numerictype  SampleTime=-1
  Constant1 : Constant  Value=false  SampleTime=-1
  Single Port RAM System : hdlsllib/HDL RAMs/Single Port RAM System  RAMType=Single port  WriteOutputValue=New data  RAMInitialValue=[gemm_wconv1(dim,:),zeros(1,4-3)]  SimulateUsing=Code generation
      settings: SourceProductBaseCode=SL
  Out1 : Outport
  wires:
  Single Port RAM System/1 -> Out1/1
  Constant/1 -> Single Port RAM System/1
  Constant1/1 -> Single Port RAM System/3
  count_Weights/1 -> Single Port RAM System/2

== system model_cnn/HDL CNN Model/Conv Layer 1/Layer 1 Mat-Vec Multiplier/Weight Storage62 ==
  count_Weights : Inport
  Constant : Constant  Value=0  OutDataTypeStr=gemm_wconv1.numerictype  SampleTime=-1
  Constant1 : Constant  Value=false  SampleTime=-1
  Single Port RAM System : hdlsllib/HDL RAMs/Single Port RAM System  RAMType=Single port  WriteOutputValue=New data  RAMInitialValue=[gemm_wconv1(dim,:),zeros(1,4-3)]  SimulateUsing=Code generation
      settings: SourceProductBaseCode=SL
  Out1 : Outport
  wires:
  Single Port RAM System/1 -> Out1/1
  Constant/1 -> Single Port RAM System/1
  Constant1/1 -> Single Port RAM System/3
  count_Weights/1 -> Single Port RAM System/2

== system model_cnn/HDL CNN Model/Conv Layer 1/Layer 1 Mat-Vec Multiplier/Weight Storage63 ==
  count_Weights : Inport
  Constant : Constant  Value=0  OutDataTypeStr=gemm_wconv1.numerictype  SampleTime=-1
  Constant1 : Constant  Value=false  SampleTime=-1
  Single Port RAM System : hdlsllib/HDL RAMs/Single Port RAM System  RAMType=Single port  WriteOutputValue=New data  RAMInitialValue=[gemm_wconv1(dim,:),zeros(1,4-3)]  SimulateUsing=Code generation
      settings: SourceProductBaseCode=SL
  Out1 : Outport
  wires:
  Single Port RAM System/1 -> Out1/1
  Constant/1 -> Single Port RAM System/1
  Constant1/1 -> Single Port RAM System/3
  count_Weights/1 -> Single Port RAM System/2

== system model_cnn/HDL CNN Model/Conv Layer 1/Layer 1 Mat-Vec Multiplier/Weight Storage7 ==
  count_Weights : Inport
  Constant : Constant  Value=0  OutDataTypeStr=gemm_wconv1.numerictype  SampleTime=-1
  Constant1 : Constant  Value=false  SampleTime=-1
  Single Port RAM System : hdlsllib/HDL RAMs/Single Port RAM System  RAMType=Single port  WriteOutputValue=New data  RAMInitialValue=[gemm_wconv1(dim,:),zeros(1,4-3)]  SimulateUsing=Code generation
      settings: SourceProductBaseCode=SL
  Out1 : Outport
  wires:
  Single Port RAM System/1 -> Out1/1
  Constant/1 -> Single Port RAM System/1
  Constant1/1 -> Single Port RAM System/3
  count_Weights/1 -> Single Port RAM System/2

== system model_cnn/HDL CNN Model/Conv Layer 1/Layer 1 Mat-Vec Multiplier/Weight Storage8 ==
  count_Weights : Inport
  Constant : Constant  Value=0  OutDataTypeStr=gemm_wconv1.numerictype  SampleTime=-1
  Constant1 : Constant  Value=false  SampleTime=-1
  Single Port RAM System : hdlsllib/HDL RAMs/Single Port RAM System  RAMType=Single port  WriteOutputValue=New data  RAMInitialValue=[gemm_wconv1(dim,:),zeros(1,4-3)]  SimulateUsing=Code generation
      settings: SourceProductBaseCode=SL
  Out1 : Outport
  wires:
  Single Port RAM System/1 -> Out1/1
  Constant/1 -> Single Port RAM System/1
  Constant1/1 -> Single Port RAM System/3
  count_Weights/1 -> Single Port RAM System/2

== system model_cnn/HDL CNN Model/Conv Layer 1/Layer 1 Mat-Vec Multiplier/Weight Storage9 ==
  count_Weights : Inport
  Constant : Constant  Value=0  OutDataTypeStr=gemm_wconv1.numerictype  SampleTime=-1
  Constant1 : Constant  Value=false  SampleTime=-1
  Single Port RAM System : hdlsllib/HDL RAMs/Single Port RAM System  RAMType=Single port  WriteOutputValue=New data  RAMInitialValue=[gemm_wconv1(dim,:),zeros(1,4-3)]  SimulateUsing=Code generation
      settings: SourceProductBaseCode=SL
  Out1 : Outport
  wires:
  Single Port RAM System/1 -> Out1/1
  Constant/1 -> Single Port RAM System/1
  Constant1/1 -> Single Port RAM System/3
  count_Weights/1 -> Single Port RAM System/2

== system model_cnn/HDL CNN Model/Conv Layer 1/Layer 1 Mat-Vec Multiplier/adder 0 ==
  In1 : Inport
  In2 : Inport  Port=2
  In3 : Inport  Port=3
  Data Type Conversion : DataTypeConversion  OutDataTypeStr=conv1_numerictype
  Multiply-Accumulate : hdlsllib/HDL Operations/Multiply-Accumulate  opMode=Streaming - using Number of Samples  initValueSetting=Dialog  initValue=0  initValueSetting2=Dialog  initValue2=0  initValueSetting3=Dialog  initValue3=0  num_samples=3  RndMeth2=Floor  RndMeth3=Floor  datatype2=Inherit: Inherit via back propagation  datatype3=accumoutdatatype1  validOut=on  endInandOut=on  startOut=on  countOut=on  dim=-1  DoSatur=off  parallel=off
      settings: SourceProductBaseCode=SL
  Terminator : Terminator
  Terminator1 : Terminator
  dataOut : Outport
  validOut : Outport  Port=2
  wires:
  ? -> validOut/1  "vectorOutValid"
  In1/1 -> Multiply-Accumulate/2
  ? -> Terminator/1  "countOut"
  Multiply-Accumulate/1 -> Data Type Conversion/1
  In3/1 -> ?
  In2/1 -> Multiply-Accumulate/1
  ? -> Terminator1/1  "validOut"
  Data Type Conversion/1 -> dataOut/1

== system model_cnn/HDL CNN Model/Conv Layer 1/Layer 1 Mat-Vec Multiplier/adder1 ==
  In1 : Inport
  In2 : Inport  Port=2
  In3 : Inport  Port=3
  Data Type Conversion : DataTypeConversion  OutDataTypeStr=conv1_numerictype
  Multiply-Accumulate : hdlsllib/HDL Operations/Multiply-Accumulate  opMode=Streaming - using Number of Samples  initValueSetting=Dialog  initValue=0  initValueSetting2=Dialog  initValue2=0  initValueSetting3=Dialog  initValue3=0  num_samples=3  RndMeth2=Floor  RndMeth3=Floor  datatype2=Inherit: Inherit via back propagation  datatype3=accumoutdatatype1  validOut=on  endInandOut=on  startOut=on  countOut=on  dim=-1  DoSatur=off  parallel=off
      settings: SourceProductBaseCode=SL
  Terminator : Terminator
  Terminator1 : Terminator
  Terminator2 : Terminator
  dataOut : Outport
  wires:
  Data Type Conversion/1 -> dataOut/1
  ? -> Terminator1/1  "validOut"
  In2/1 -> Multiply-Accumulate/1
  In3/1 -> ?
  Multiply-Accumulate/1 -> Data Type Conversion/1
  ? -> Terminator/1  "countOut"
  In1/1 -> Multiply-Accumulate/2
  ? -> Terminator2/1  "vectorOutValid"

== system model_cnn/HDL CNN Model/Conv Layer 1/Layer 1 Mat-Vec Multiplier/adder10 ==
  In1 : Inport
  In2 : Inport  Port=2
  In3 : Inport  Port=3
  Data Type Conversion : DataTypeConversion  OutDataTypeStr=conv1_numerictype
  Multiply-Accumulate : hdlsllib/HDL Operations/Multiply-Accumulate  opMode=Streaming - using Number of Samples  initValueSetting=Dialog  initValue=0  initValueSetting2=Dialog  initValue2=0  initValueSetting3=Dialog  initValue3=0  num_samples=3  RndMeth2=Floor  RndMeth3=Floor  datatype2=Inherit: Inherit via back propagation  datatype3=accumoutdatatype1  validOut=on  endInandOut=on  startOut=on  countOut=on  dim=-1  DoSatur=off  parallel=off
      settings: SourceProductBaseCode=SL
  Terminator : Terminator
  Terminator1 : Terminator
  Terminator2 : Terminator
  dataOut : Outport
  wires:
  Data Type Conversion/1 -> dataOut/1
  ? -> Terminator1/1  "validOut"
  In2/1 -> Multiply-Accumulate/1
  In3/1 -> ?
  Multiply-Accumulate/1 -> Data Type Conversion/1
  ? -> Terminator/1  "countOut"
  In1/1 -> Multiply-Accumulate/2
  ? -> Terminator2/1  "vectorOutValid"

== system model_cnn/HDL CNN Model/Conv Layer 1/Layer 1 Mat-Vec Multiplier/adder11 ==
  In1 : Inport
  In2 : Inport  Port=2
  In3 : Inport  Port=3
  Data Type Conversion : DataTypeConversion  OutDataTypeStr=conv1_numerictype
  Multiply-Accumulate : hdlsllib/HDL Operations/Multiply-Accumulate  opMode=Streaming - using Number of Samples  initValueSetting=Dialog  initValue=0  initValueSetting2=Dialog  initValue2=0  initValueSetting3=Dialog  initValue3=0  num_samples=3  RndMeth2=Floor  RndMeth3=Floor  datatype2=Inherit: Inherit via back propagation  datatype3=accumoutdatatype1  validOut=on  endInandOut=on  startOut=on  countOut=on  dim=-1  DoSatur=off  parallel=off
      settings: SourceProductBaseCode=SL
  Terminator : Terminator
  Terminator1 : Terminator
  Terminator2 : Terminator
  dataOut : Outport
  wires:
  Data Type Conversion/1 -> dataOut/1
  ? -> Terminator1/1  "validOut"
  In2/1 -> Multiply-Accumulate/1
  In3/1 -> ?
  Multiply-Accumulate/1 -> Data Type Conversion/1
  ? -> Terminator/1  "countOut"
  In1/1 -> Multiply-Accumulate/2
  ? -> Terminator2/1  "vectorOutValid"

== system model_cnn/HDL CNN Model/Conv Layer 1/Layer 1 Mat-Vec Multiplier/adder12 ==
  In1 : Inport
  In2 : Inport  Port=2
  In3 : Inport  Port=3
  Data Type Conversion : DataTypeConversion  OutDataTypeStr=conv1_numerictype
  Multiply-Accumulate : hdlsllib/HDL Operations/Multiply-Accumulate  opMode=Streaming - using Number of Samples  initValueSetting=Dialog  initValue=0  initValueSetting2=Dialog  initValue2=0  initValueSetting3=Dialog  initValue3=0  num_samples=3  RndMeth2=Floor  RndMeth3=Floor  datatype2=Inherit: Inherit via back propagation  datatype3=accumoutdatatype1  validOut=on  endInandOut=on  startOut=on  countOut=on  dim=-1  DoSatur=off  parallel=off
      settings: SourceProductBaseCode=SL
  Terminator : Terminator
  Terminator1 : Terminator
  Terminator2 : Terminator
  dataOut : Outport
  wires:
  Data Type Conversion/1 -> dataOut/1
  ? -> Terminator1/1  "validOut"
  In2/1 -> Multiply-Accumulate/1
  In3/1 -> ?
  Multiply-Accumulate/1 -> Data Type Conversion/1
  ? -> Terminator/1  "countOut"
  In1/1 -> Multiply-Accumulate/2
  ? -> Terminator2/1  "vectorOutValid"

== system model_cnn/HDL CNN Model/Conv Layer 1/Layer 1 Mat-Vec Multiplier/adder13 ==
  In1 : Inport
  In2 : Inport  Port=2
  In3 : Inport  Port=3
  Data Type Conversion : DataTypeConversion  OutDataTypeStr=conv1_numerictype
  Multiply-Accumulate : hdlsllib/HDL Operations/Multiply-Accumulate  opMode=Streaming - using Number of Samples  initValueSetting=Dialog  initValue=0  initValueSetting2=Dialog  initValue2=0  initValueSetting3=Dialog  initValue3=0  num_samples=3  RndMeth2=Floor  RndMeth3=Floor  datatype2=Inherit: Inherit via back propagation  datatype3=accumoutdatatype1  validOut=on  endInandOut=on  startOut=on  countOut=on  dim=-1  DoSatur=off  parallel=off
      settings: SourceProductBaseCode=SL
  Terminator : Terminator
  Terminator1 : Terminator
  Terminator2 : Terminator
  dataOut : Outport
  wires:
  Data Type Conversion/1 -> dataOut/1
  ? -> Terminator1/1  "validOut"
  In2/1 -> Multiply-Accumulate/1
  In3/1 -> ?
  Multiply-Accumulate/1 -> Data Type Conversion/1
  ? -> Terminator/1  "countOut"
  In1/1 -> Multiply-Accumulate/2
  ? -> Terminator2/1  "vectorOutValid"
